simulink model "testGp"  (R2018b)
settings: Solver=VariableStepAuto  StartTime=0.0  StopTime=10.0  RelTol=1e-3
libraries: gaussianProcess_ul x1
settings Model: Creator=asiddiq2  LastModifiedBy=asiddiq2

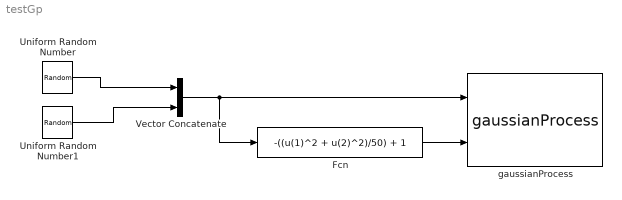
== system testGp ==
  Fcn : Fcn  Expr=-((u(1)^2 + u(2)^2)/50) + 1
  Uniform Random Number : UniformRandomNumber  Minimum=-5  Maximum=5  Seed=randi(1000)  SampleTime=0.1
  Uniform Random Number1 : UniformRandomNumber  Minimum=-5  Maximum=5  Seed=randi(1000)  SampleTime=0.1
  Vector Concatenate : Concatenate
  gaussianProcess : gaussianProcess_ul/gaussianProcess  dt=1
  wires:
  Fcn/1 -> gaussianProcess/2
  Uniform Random Number/1 -> Vector Concatenate/1
  Uniform Random Number1/1 -> Vector Concatenate/2
  Vector Concatenate/1 -> Fcn/1, gaussianProcess/1
